simulink model "Question1_system"  (R2020b)
settings: Solver=ode45  StartTime=0.0  StopTime=10.0  MaxStep=0.001  RelTol=1e-3
values from neighbouring files (symbols this model uses):
  b = 50    [Question1_code.m]
  h2r = 2*pi    (= 6.28318530718)    [Question1_code.m]
  k1 = 50    [Question1_code.m]
  m1 = 100    [Question1_code.m]
settings Model: Creator=sneha  LastModifiedBy=sneha

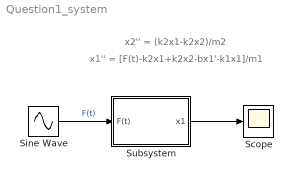
== system Question1_system ==
  note: x1'' = [F(t)-k2x1+k2x2-bx1'-k1x1]/m1
  note: x2'' = (k2x1-k2x2)/m2
  Scope : Scope
  Sine Wave : Sin  Amplitude=2  Frequency=10*h2r  SampleTime=0
  Subsystem : Subsystem  mask{m2=0, k12=0}
      mask prompts: m2 "mass2"; k12 "spring constant 2"
  wires:
  Sine Wave/1 -> Subsystem/1(F(t))  "F(t)"
  Subsystem/1(x1) -> Scope/1

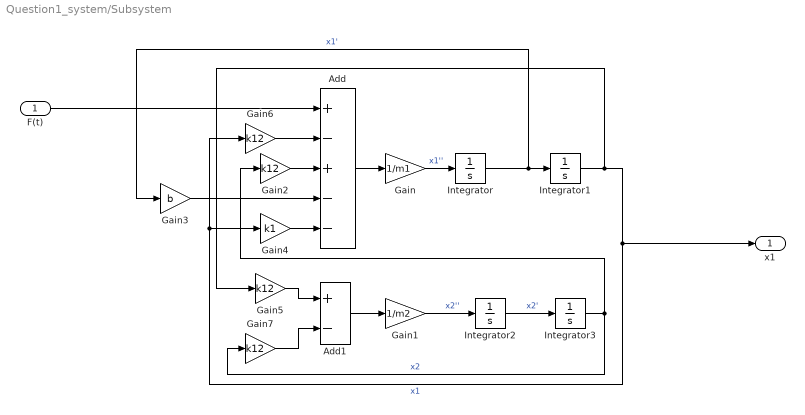
== system Question1_system/Subsystem ==
  F(t) : Inport
  Add : Sum  Inputs=+-+--
  Add1 : Sum  Inputs=+-
  Gain : Gain  Gain=1/m1
  Gain1 : Gain  Gain=1/m2
  Gain{2,5..7} (4 alike) : Gain  Gain=k12
  Gain3 : Gain  Gain=b
  Gain4 : Gain  Gain=k1
  Integrator{,1..3} (4 alike) : Integrator
  x1 : Outport
  wires:
  Integrator/1 -> Gain3/1, Integrator1/1  "x1'"
  Gain6/1 -> Add/2
  Add/1 -> Gain/1
  Gain2/1 -> Add/3
  Integrator3/1 -> Gain2/1, Gain7/1  "x2"
  Gain7/1 -> Add1/2
  Add1/1 -> Gain1/1
  Gain5/1 -> Add1/1
  Gain4/1 -> Add/5
  Gain3/1 -> Add/4
  Integrator1/1 -> Gain5/1, x1/1, Gain6/1, Gain4/1  "x1"
  Gain/1 -> Integrator/1  "x1''"
  Integrator2/1 -> Integrator3/1  "x2'"
  Gain1/1 -> Integrator2/1  "x2''"
  F(t)/1 -> Add/1
